simulink model "ssc_lithium_cell_1RC"  (Simulink 7.6)
settings: Solver=ode15s  StartTime=0.0  StopTime=40000  RelTol=1e-3
PreLoadFcn:
  | ssc_lithium_cell_1RC_ini
values from neighbouring files (symbols this model uses):
  C1_LUT = [ ... (first row only)    [ssc_lithium_cell_1RC_ini.m]
  Capacity_LUT = [ ... (first row only)    [ssc_lithium_cell_1RC_ini.m]
  cell_Cp_heat = cell_rho_Cp * cell_volume    (= 810.5328)    [ssc_lithium_cell_1RC_ini.m]
  cell_mass = 1    [ssc_lithium_cell_1RC_ini.m]
  Em_LUT = [ ... (first row only)    [ssc_lithium_cell_1RC_ini.m]
  Qe_init = 15.6845    [ssc_lithium_cell_1RC_ini.m]
  R0_LUT = [ ... (first row only)    [ssc_lithium_cell_1RC_ini.m]
  R1_LUT = [ ... (first row only)    [ssc_lithium_cell_1RC_ini.m]
  SOC_LUT = [0 0.1 0.25 0.5 0.75 0.9 1]'    [ssc_lithium_cell_1RC_ini.m]
  T_init = 20 + 273.15    (= 293.15)    [ssc_lithium_cell_1RC_ini.m]
  Temperature_LUT = [5 20 40] + 273.15    [ssc_lithium_cell_1RC_ini.m]
undefined symbols (not defined in the file or in its folder): sigbuilder_block
libraries: fl_lib x17, nesl_utility x6, LiBatteryElements_lib x4
Description:
  | Lithium Battery Cell - 1 RC Branch Equivalent Circuit
  | 
  | This demo implements a model of a lithium cell using the Simscape language to implement the elements of an equivalent circuit model with one RC branch. For the defining equations and their validation, see T. Huria, M. Ceraolo, J. Gazzarri, R. Jackey. "High Fidelity Electrical Model with Thermal Dependence for Characterization and Simulation of High Power Lithium Battery Cells," IEEE International Electric Vehicle Conference, March 2012.
  | 
  | A simple thermal model is used to model battery temperature. It is assumed that cooling is primarily via convection, and that heating is primarily from battery internal resistance. A battery pack can be modeled by connecting multiple copies of the battery cell block in series.
  | 
  | Copyright 2012 The MathWorks, Inc.
settings Model: Creator=MathWorks  LastModifiedBy=rjackey
settings DataIOCC: SaveOutput=off  SaveTime=off
settings DebuggingCC: SolverPrmCheckMsg=none  StrictBusMsg=Warning

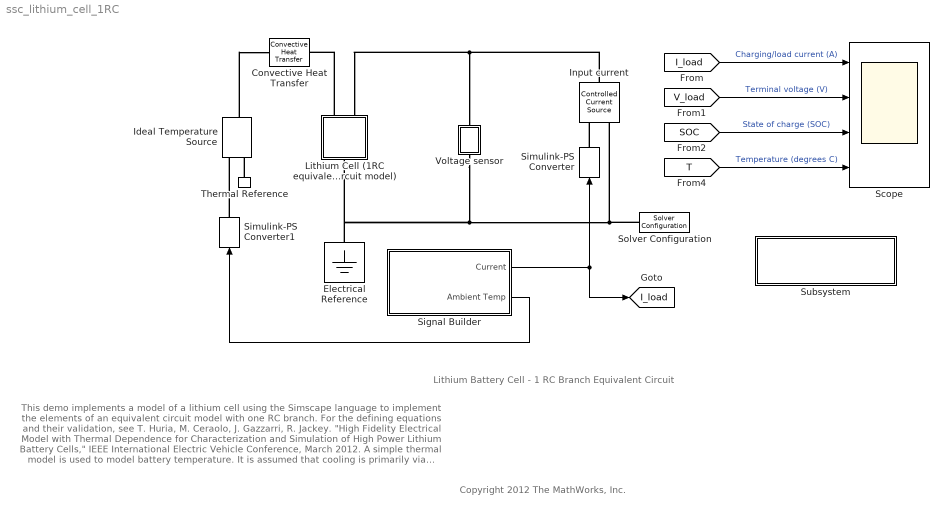
== system ssc_lithium_cell_1RC ==
  note: Lithium Battery Cell - 1 RC Branch Equivalent Circuit
  note: This demo implements a model of a lithium cell using the Simscape language to implement the elements of an equivalent circuit model with one
      | RC branch. For the defining equations and their validation, see T. Huria, M. Ceraolo, J. Gazzarri, R. Jackey. "High Fidelity Electrical Model with
      | Thermal Dependence for Characterization and Simulation of High Power Lithium Battery Cells," IEEE International Electric Vehicle Conference,
      | March 2012. A simple thermal model is used to model battery temperature. It is assumed that cooling is primarily via convection, and that heating
      | is primarily from internal resistance. A battery pack can be modeled by connecting multiple copies of the battery cell block in series.
  note: Copyright 2012 The MathWorks, Inc.
  Convective Heat Transfer : fl_lib/Thermal/Thermal Elements/Convective Heat Transfer  DialogController=NetworkEngine.DynNeDlgSource  SystemSampleTime=-1  area=cell_area m^2  heat_tr_coeff=h_conv W/(m^2 * K)  Q_Log=off  T_Log=off  LocalVarNames=|heat_flow|temperature_diff  LocalVarDescs=|Heat flow (J/s)|Temperature difference (K)  LocalVarLogging=[0 0]
  Electrical Reference : fl_lib/Electrical/Electrical Elements/Electrical Reference  DialogController=NetworkEngine.DynNeDlgSource  SystemSampleTime=-1  i_Log=off  LocalVarNames=|i  LocalVarDescs=|i  LocalVarLogging=[]
  Ideal Temperature Source : fl_lib/Thermal/Thermal Sources/Ideal Temperature Source  DialogController=NetworkEngine.DynNeDlgSource  SystemSampleTime=-1  Q_Log=off  T_Log=off  LocalVarNames=|heat_flow|T_differential  LocalVarDescs=|Heat flow rate through the source (J/s)|Temperature differential across the source (K)  LocalVarLogging=[0 0]
  Input current : fl_lib/Electrical/Electrical Sources/Controlled Current Source  DialogController=NetworkEngine.DynNeDlgSource  SystemSampleTime=-1  i_Log=off  v_Log=off  LocalVarNames=|current|voltage|power  LocalVarDescs=|Current (A)|Voltage (V)|Power (W)  LocalVarLogging=[0 0 0]
  Lithium Cell (1RC equivalent circuit model) : Subsystem  mask{Qe_init=Qe_init, T_init=T_init, Capacity_LUT=Capacity_LUT, Em_LUT=Em_LUT, R0_LUT=R0_LUT, R1_LUT=R1_LUT, C1_LUT=C1_LUT, cell_mass=cell_mass, cell_Cp_heat=cell_Cp_heat, SOC_LUT=SOC_LUT, Temperature_LUT=Temperature_LUT}
      mask prompts: Qe_init "Initial Charge Deficit (A*hr)"; T_init "Initial Cell Temperature (K)"; Capacity_LUT "Capacity (A*hr, 1xN table)"; Em_LUT "Em Open-Circuit Voltage (MxN table)"; R0_LUT "R0: Terminal Resistance (Ohms, MxN table)"; R1_LUT "R1 Resistance (Ohms, MxN table)"; C1_LUT "C1 Capacitance (Farads, MxN table)"; cell_mass "Cell Mass (kg)"; cell_Cp_heat "Cell Specific Heat (J/kg/K)"; SOC_LUT "SOC Table Breakpoints (Mx1 array)"; Temperature_LUT "Temperature Table Breakpoints(K, 1xN array)"
      mask TabNameString: Initial Conditions,Initial Conditions,Electrical,Electrical,Electrical,Electrical,Electrical,Thermal,Thermal,Table Breakpoints,Table Breakpoints
      mask Display:
      | image(imread('battery.jpg'))
      | color('red')
      | port_label('LConn',1,'H')
      | port_label('LConn',2,'+')
      | port_label('RConn',1,'-')
  Scope : Scope  NumInputPorts=4
      settings: TimeRange=40000  YMin=-35~3~0~20  YMax=35~4.5~1~35
  Signal Builder : Subsystem  Tag=STV Subsys  LoadFcn=sigbuilder_block('load');  StartFcn=sigbuilder_block('start');  StopFcn=sigbuilder_block('stop');  ClipboardFcn=sigbuilder_block('clipboard');  mask(Sigbuilder block){}
      mask help: Simulink:masks:SigbuilderBlock_MD
      mask init:
      | if ~strcmp(get_param(bdroot(gcbh),'SimulationStatus'),'stopped') tuvar = sigbuilder_block('maskInit'); end
      settings: CopyFcn=sigbuilder_block('copy');  DeleteFcn=sigbuilder_block('delete');  ModelCloseFcn=sigbuilder_block('modelClose');  PreSaveFcn=sigbuilder_block('preSave');  NameChangeFcn=sigbuilder_block('namechange');  OpenFcn=sigbuilder_block('open',[62.25 82.5 550.5 303 ]);  CloseFcn=sigbuilder_block('close');
      mask Display: plot(0,0,100,100,[10,10,40,40,10],[80,20,20,80,80],[40,10],[50,50], [40,27,10],[65,72,56],[40,25,25,10],[28,28,43,43]);
  Simulink-PS Converter : nesl_utility/Simulink-PS Converter  DialogController=NetworkEngine.DynNeUtilDlgSource  SystemSampleTime=-1  PhysicalDomain=network_engine_domain  LeftPortType=input  RightPortType=output  SubClassName=ps_input  Unit=A  AffineConversion=on  InputFilterTimeConstant=.001  UdotUserProvided=0
  Simulink-PS Converter1 : nesl_utility/Simulink-PS Converter  DialogController=NetworkEngine.DynNeUtilDlgSource  SystemSampleTime=-1  PhysicalDomain=network_engine_domain  LeftPortType=input  RightPortType=output  SubClassName=ps_input  Unit=C  AffineConversion=on  InputFilterTimeConstant=.001  UdotUserProvided=0
  Solver Configuration : nesl_utility/Solver Configuration  DialogController=NetworkEngine.DynNeUtilDlgSource  SystemSampleTime=-1  PhysicalDomain=network_engine_domain  LeftPortType=input  RightPortType=generic  SubClassName=solver  Accelerate=off  Profile=off  ResidualTolerance=1e-9  MaxNonlinIter=3  MaxModeIter=2  DoFixedCost=off  UseLocalSampling=off  DoDC=off  LinearAlgebra=Sparse  LocalSolverSampleTime=.001  LocalSolverChoice=NE_BACKWARD_EULER_ADVANCER  UseLocalSolver=off
  Subsystem : Subsystem
      settings: OpenFcn=open('LiBatteryElements_lib.mdl')
      mask Display: disp('Open the custom\n library used by the\n Lithium Cell block')
  Thermal Reference : fl_lib/Thermal/Thermal Elements/Thermal Reference  DialogController=NetworkEngine.DynNeDlgSource  SystemSampleTime=-1  Q_Log=off  LocalVarNames=|Q  LocalVarDescs=|Q  LocalVarLogging=[]
  Voltage sensor : Subsystem
  tag scope: I_load=global
  wires:
  [SOC] -> Scope/3  "State of charge (SOC)"
  [T] -> Scope/4  "Temperature (degrees C)"
  [I_load] -> Scope/1  "Charging/load current (A)"
  [V_load] -> Scope/2  "Terminal voltage (V)"
  Signal Builder/2(Ambient Temp) -> Simulink-PS Converter1/1
  Signal Builder/1(Current) -> Simulink-PS Converter/1, [I_load]
  connections:
  Electrical Reference/LConn1 -- Lithium Cell (1RC equivalent circuit model)/RConn1 -- Solver Configuration/RConn1 -- Input current/RConn2 -- Voltage sensor/RConn1
  Input current/LConn1 -- Lithium Cell (1RC equivalent circuit model)/LConn2 -- Voltage sensor/LConn1
  Thermal Reference/LConn1 -- Ideal Temperature Source/RConn2
  Ideal Temperature Source/LConn1 -- Convective Heat Transfer/LConn1
  Lithium Cell (1RC equivalent circuit model)/LConn1 -- Convective Heat Transfer/RConn1
  Simulink-PS Converter/RConn1 -- Input current/RConn1
  Simulink-PS Converter1/RConn1 -- Ideal Temperature Source/RConn1

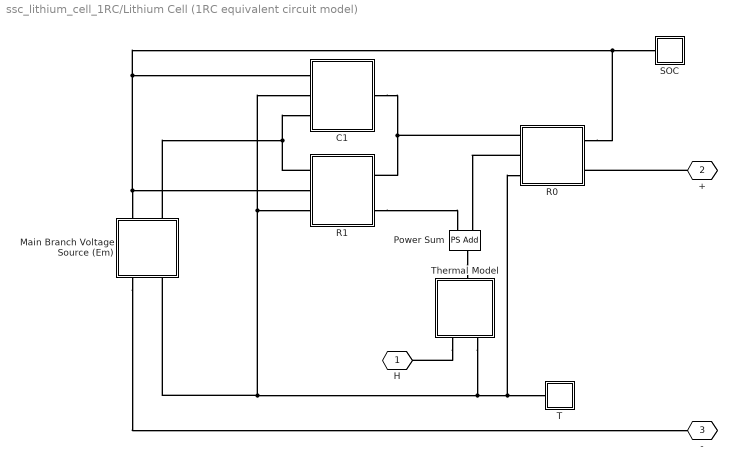
== system ssc_lithium_cell_1RC/Lithium Cell (1RC equivalent circuit model) ==
  " SOC " : Subsystem
  C1 : Subsystem
  Main Branch Voltage Source (Em) : Subsystem
  Power Sum : fl_lib/Physical Signals/Functions/PS Add  DialogController=NetworkEngine.DynNeDlgSource  SystemSampleTime=-1  LocalVarLogging=[]
  R0 : Subsystem
  R1 : Subsystem
  T : Subsystem
  Thermal Model : Subsystem
  H : PMIOPort  Tag=PMCPort  Port=1  Side=Left
  + : PMIOPort  Tag=PMCPort  Port=2  Side=Left
  - : PMIOPort  Tag=PMCPort  Port=3  Side=Right
  connections:
  Main Branch Voltage Source (Em)/LConn1 -- R1/LConn2 -- C1/LConn1 -- " SOC "/LConn1 -- R0/RConn1
  Thermal Model/RConn1 -- H/RConn1
  Main Branch Voltage Source (Em)/RConn1 -- -/RConn1
  +/RConn1 -- R0/RConn2
  R1/LConn1 -- C1/LConn3 -- Main Branch Voltage Source (Em)/LConn2
  R1/RConn2 -- Power Sum/LConn2
  R0/LConn2 -- Power Sum/LConn1
  Main Branch Voltage Source (Em)/RConn2 -- C1/LConn2 -- R1/LConn3 -- Thermal Model/RConn2 -- T/LConn1 -- R0/LConn3
  Power Sum/RConn1 -- Thermal Model/LConn1
  R0/LConn1 -- R1/RConn1 -- C1/RConn1

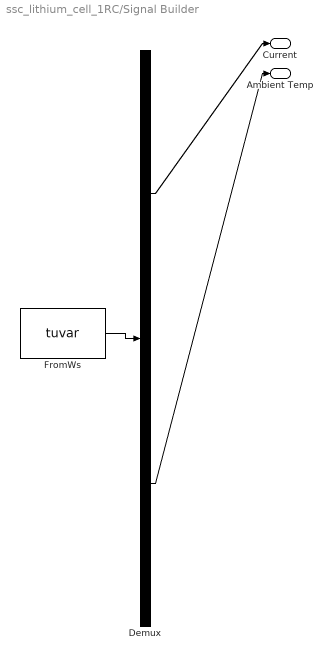
== system ssc_lithium_cell_1RC/Signal Builder ==
  Demux : Demux  Tag=STV Demux  Outputs=2
  FromWs : FromWorkspace  Tag=STV FromWs  VariableName=tuvar  SampleTime=0  SigBuilderData=DataTag0  VnvData=DataTag1
      SigBuilderData=|
      | common.afterFinalStr = 'Extrapolate'
      | common.sampleTime = 0
      | dataSet(1).timeRange = [0 40000]
      | dataSet(1).name = 'Pulse'
      | dataSet(2).timeRange = [0 40000]
      | dataSet(2).name = 'Constant'
      | sbobj.Name = 'Signal Builder'
      | sbobj.Groups(1).Name = 'Pulse'
      | sbobj.Groups(1).Signals(1).Name = 'Current'
      | sbobj.Groups(1).Signals(1).XData = [0 300 300 2100 2100 3600 3600 3960 3960 7200 7200 7560 7560 10800 10800 11160 11160 14400 14400 14760 14760 18000 18000 18360 18360 21600 21600 21960 21960 25200 25200 25560 25560 28800 28800 29160 29160 32400 32400 32760 32760 36000 36000 36360 36360 40000]
      | sbobj.Groups(1).Signals(1).YData = [0 0 31.5 31.5 0 0 -27.625 -27.625 0 0 -27.625 -27.625 0 0 -27.625 -27.625 0 0 -27.625 -27.625 0 0 -27.625 -27.625 0 0 -27.625 -27.625 0 0 -27.625 -27.625 0 0 -27.625 -27.625 0 0 -27.625 -27.625 0 0 -27.625 -27.625 0 0]
      | sbobj.Groups(1).Signals(2).Name = 'Ambient Temp'
      | sbobj.Groups(1).Signals(2).XData = [0 300 300 2100 2100 3600 3600 3960 3960 7200 7200 7560 7560 10800 10800 11160 11160 14400 14400 14760 14760 18000 18000 18360 18360 21600 21600 21960 21960 25200 25200 25560 25560 28800 28800 29160 29160 32400 32400 32760 32760 36000 36000 36360 36360 40000]
      | sbobj.Groups(1).Signals(2).YData = [20 20 20 20 20 20 20 20 20 20 20 20 20 20 20 20 20 20 20 20 20 20 20 20 20 20 20 20 20 20 20 20 20 20 20 20 20 20 20 20 20 20 20 20 20 20]
      | sbobj.Groups(1).TimeRange = [0 40000]
      | sbobj.Groups(2).Name = 'Constant'
      | sbobj.Groups(2).Signals(1).Name = 'Current'
      | sbobj.Groups(2).Signals(1).XData = [0 360 360 9100 9100 11800 11800 28200 33800 40000]
      | sbobj.Groups(2).Signals(1).YData = [0 0 -5 -5 0 0 5 5 0 0]
      | sbobj.Groups(2).Signals(2).Name = 'Ambient Temp'
      | sbobj.Groups(2).Signals(2).XData = [0 360 360 9100 9100 11800 11800 28200 33800 40000]
      | sbobj.Groups(2).Signals(2).YData = [20 20.09 20.09 22.275 22.275 22.95 22.95 27.05 28.45 30]
      | sbobj.Groups(2).TimeRange = [0 40000]
  Current : Outport
  Ambient Temp : Outport  Tag=STV Outport  Port=2
  wires:
  FromWs/1 -> Demux/1
  Demux/1 -> Current/1
  Demux/2 -> Ambient Temp/1

== system ssc_lithium_cell_1RC/Subsystem ==

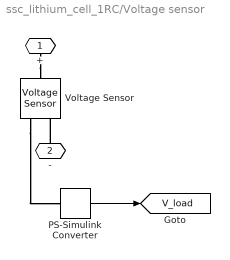
== system ssc_lithium_cell_1RC/Voltage sensor ==
  PS-Simulink Converter : nesl_utility/PS-Simulink Converter  DialogController=NetworkEngine.DynNeUtilDlgSource  SystemSampleTime=-1  PhysicalDomain=network_engine_domain  LeftPortType=input  RightPortType=output  SubClassName=ps_output  Unit=V  AffineConversion=off
  Voltage Sensor : fl_lib/Electrical/Electrical Sensors/Voltage Sensor  DialogController=NetworkEngine.DynNeDlgSource  SystemSampleTime=-1  i1_Log=off  v1_Log=off  LocalVarNames=|i1|v1  LocalVarDescs=|i1|v1  LocalVarLogging=[]
  + : PMIOPort  Port=1  Side=Left
  - : PMIOPort  Port=2  Side=Right
  tag scope: V_load=global
  wires:
  PS-Simulink Converter/1 -> [V_load]
  connections:
  Voltage Sensor/RConn1 -- PS-Simulink Converter/LConn1
  +/RConn1 -- Voltage Sensor/LConn1
  -/RConn1 -- Voltage Sensor/RConn2

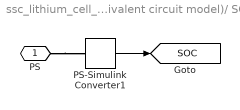
== system ssc_lithium_cell_1RC/Lithium Cell (1RC equivalent circuit model)/ SOC  ==
  PS-Simulink Converter1 : nesl_utility/PS-Simulink Converter  DialogController=NetworkEngine.DynNeUtilDlgSource  SystemSampleTime=-1  PhysicalDomain=network_engine_domain  LeftPortType=input  RightPortType=output  SubClassName=ps_output  Unit=1  AffineConversion=off
  PS : PMIOPort  Port=1  Side=Left
  tag scope: SOC=global
  wires:
  PS-Simulink Converter1/1 -> [SOC]
  connections:
  PS/RConn1 -- PS-Simulink Converter1/LConn1

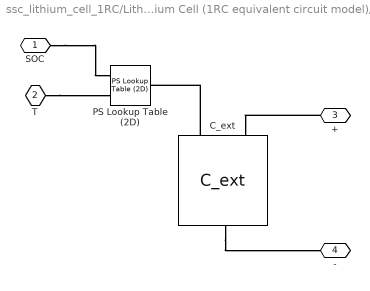
== system ssc_lithium_cell_1RC/Lithium Cell (1RC equivalent circuit model)/C1 ==
  C_ext : LiBatteryElements_lib/C_ext  DialogController=NetworkEngine.DynNeDlgSource  SystemSampleTime=-1  v0=0 V  Cmin=1e-6 F  i_Log=off  v_Log=off  LocalVarNames=|i|v  LocalVarDescs=|i|v  LocalVarLogging=[0 0]
  PS Lookup Table (2D) : fl_lib/Physical Signals/Lookup Tables/PS Lookup Table (2D)  DialogController=NetworkEngine.DynNeDlgSource  SystemSampleTime=-1  x_t=SOC_LUT  y_t=Temperature_LUT  z_t=C1_LUT  interp_method=1  extrap_method=1  dbg=0  LocalVarLogging=[]
  SOC : PMIOPort  Port=1  Side=Left
  T : PMIOPort  Port=2  Side=Left
  + : PMIOPort  Port=3  Side=Left
  - : PMIOPort  Port=4  Side=Right
  connections:
  SOC/RConn1 -- PS Lookup Table (2D)/LConn1
  T/RConn1 -- PS Lookup Table (2D)/LConn2
  C_ext/LConn2 -- PS Lookup Table (2D)/RConn1
  C_ext/RConn1 -- -/RConn1
  +/RConn1 -- C_ext/LConn1

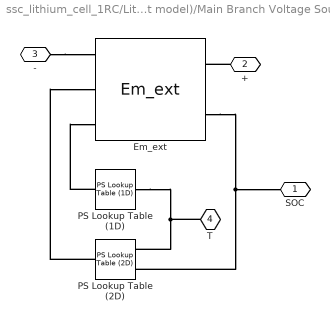
== system ssc_lithium_cell_1RC/Lithium Cell (1RC equivalent circuit model)/Main Branch Voltage Source (Em) ==
  Em_ext : LiBatteryElements_lib/Em_ext  DialogController=NetworkEngine.DynNeDlgSource  SystemSampleTime=-1  Qinit=Qe_init hr*A  i_Log=off  v_Log=off  Qe_Log=off  LocalVarNames=|i|v|Qe  LocalVarDescs=|i|v|Extracted charge  LocalVarLogging=[0 0 0]
  PS Lookup Table (1D) : fl_lib/Physical Signals/Lookup Tables/PS Lookup Table (1D)  DialogController=NetworkEngine.DynNeDlgSource  SystemSampleTime=-1  x_t=Temperature_LUT  y_t=Capacity_LUT  interp_method=1  extrap_method=1  dbg=0  LocalVarLogging=[]
  PS Lookup Table (2D) : fl_lib/Physical Signals/Lookup Tables/PS Lookup Table (2D)  DialogController=NetworkEngine.DynNeDlgSource  SystemSampleTime=-1  x_t=SOC_LUT  y_t=Temperature_LUT  z_t=Em_LUT  interp_method=1  extrap_method=1  dbg=0  LocalVarLogging=[]
  SOC : PMIOPort  Port=1  Side=Left
  + : PMIOPort  Port=2  Side=Left
  - : PMIOPort  Port=3  Side=Right
  T : PMIOPort  Port=4  Side=Right
  connections:
  -/RConn1 -- Em_ext/RConn1
  +/RConn1 -- Em_ext/LConn1
  Em_ext/LConn2 -- SOC/RConn1 -- PS Lookup Table (2D)/LConn1
  PS Lookup Table (2D)/RConn1 -- Em_ext/RConn2
  PS Lookup Table (1D)/LConn1 -- PS Lookup Table (2D)/LConn2 -- T/RConn1
  PS Lookup Table (1D)/RConn1 -- Em_ext/RConn3

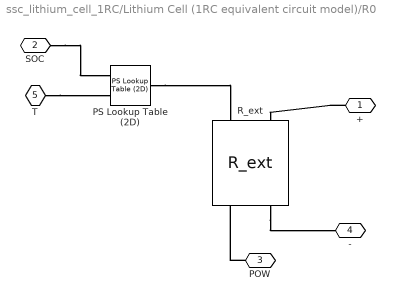
== system ssc_lithium_cell_1RC/Lithium Cell (1RC equivalent circuit model)/R0 ==
  PS Lookup Table (2D) : fl_lib/Physical Signals/Lookup Tables/PS Lookup Table (2D)  DialogController=NetworkEngine.DynNeDlgSource  SystemSampleTime=-1  x_t=SOC_LUT  y_t=Temperature_LUT  z_t=R0_LUT  interp_method=1  extrap_method=1  dbg=0  LocalVarLogging=[]
  R_ext : LiBatteryElements_lib/R_ext  DialogController=NetworkEngine.DynNeDlgSource  SystemSampleTime=-1  Rmin=0 Ohm  i_Log=off  v_Log=off  LocalVarNames=|i|v  LocalVarDescs=|i|v  LocalVarLogging=[0 0]
  + : PMIOPort  Port=1  Side=Left
  SOC : PMIOPort  Port=2  Side=Right
  POW : PMIOPort  Port=3  Side=Left
  - : PMIOPort  Port=4  Side=Right
  T : PMIOPort  Port=5  Side=Left
  connections:
  T/RConn1 -- PS Lookup Table (2D)/LConn2
  +/RConn1 -- R_ext/LConn1
  R_ext/RConn1 -- -/RConn1
  POW/RConn1 -- R_ext/RConn2
  PS Lookup Table (2D)/RConn1 -- R_ext/LConn2
  SOC/RConn1 -- PS Lookup Table (2D)/LConn1

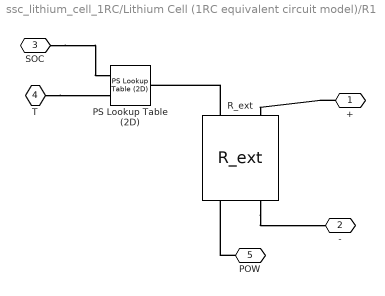
== system ssc_lithium_cell_1RC/Lithium Cell (1RC equivalent circuit model)/R1 ==
  PS Lookup Table (2D) : fl_lib/Physical Signals/Lookup Tables/PS Lookup Table (2D)  DialogController=NetworkEngine.DynNeDlgSource  SystemSampleTime=-1  x_t=SOC_LUT  y_t=Temperature_LUT  z_t=R1_LUT  interp_method=1  extrap_method=1  dbg=0  LocalVarLogging=[]
  R_ext : LiBatteryElements_lib/R_ext  DialogController=NetworkEngine.DynNeDlgSource  SystemSampleTime=-1  Rmin=0 Ohm  i_Log=off  v_Log=off  LocalVarNames=|i|v  LocalVarDescs=|i|v  LocalVarLogging=[0 0]
  + : PMIOPort  Port=1  Side=Left
  - : PMIOPort  Port=2  Side=Right
  SOC : PMIOPort  Port=3  Side=Left
  T : PMIOPort  Port=4  Side=Left
  POW : PMIOPort  Port=5  Side=Right
  connections:
  SOC/RConn1 -- PS Lookup Table (2D)/LConn1
  T/RConn1 -- PS Lookup Table (2D)/LConn2
  R_ext/LConn2 -- PS Lookup Table (2D)/RConn1
  POW/RConn1 -- R_ext/RConn2
  R_ext/RConn1 -- -/RConn1
  +/RConn1 -- R_ext/LConn1

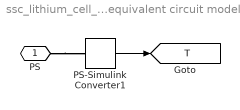
== system ssc_lithium_cell_1RC/Lithium Cell (1RC equivalent circuit model)/T ==
  PS-Simulink Converter1 : nesl_utility/PS-Simulink Converter  DialogController=NetworkEngine.DynNeUtilDlgSource  SystemSampleTime=-1  PhysicalDomain=network_engine_domain  LeftPortType=input  RightPortType=output  SubClassName=ps_output  Unit=C  AffineConversion=on
  PS : PMIOPort  Port=1  Side=Left
  tag scope: T=global
  wires:
  PS-Simulink Converter1/1 -> [T]
  connections:
  PS/RConn1 -- PS-Simulink Converter1/LConn1

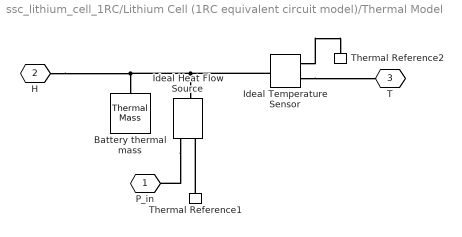
== system ssc_lithium_cell_1RC/Lithium Cell (1RC equivalent circuit model)/Thermal Model ==
  Battery thermal mass : fl_lib/Thermal/Thermal Elements/Thermal Mass  DialogController=NetworkEngine.DynNeDlgSource  SystemSampleTime=-1  mass=cell_mass kg  sp_heat=cell_Cp_heat J/kg/K  init_temp=T_init K  Q_Log=off  LocalVarNames=|heat_flow|temperature  LocalVarDescs=|Heat flow (J/s)|Mass temperature (K)  LocalVarLogging=[0 0]
  Ideal Temperature Sensor : fl_lib/Thermal/Thermal Sensors/Ideal Temperature Sensor  DialogController=NetworkEngine.DynNeDlgSource  SystemSampleTime=-1  Qs_Log=off  Ts_Log=off  LocalVarNames=|Qs|Ts  LocalVarDescs=|Qs|Ts  LocalVarLogging=[]
  Ideal Heat Flow Source : fl_lib/Thermal/Thermal Sources/Ideal Heat Flow Source  DialogController=NetworkEngine.DynNeDlgSource  SystemSampleTime=-1  Q_Log=off  T_Log=off  LocalVarNames=|heat_flow|T_differential  LocalVarDescs=|Heat flow through the source (J/s)|Temperature differential across the source (K)  LocalVarLogging=[0 0]
  Thermal Reference1 : fl_lib/Thermal/Thermal Elements/Thermal Reference  DialogController=NetworkEngine.DynNeDlgSource  SystemSampleTime=-1  Q_Log=off  LocalVarNames=|Q  LocalVarDescs=|Q  LocalVarLogging=[]
  Thermal Reference2 : fl_lib/Thermal/Thermal Elements/Thermal Reference  DialogController=NetworkEngine.DynNeDlgSource  SystemSampleTime=-1  Q_Log=off  LocalVarNames=|Q  LocalVarDescs=|Q  LocalVarLogging=[]
  P_in : PMIOPort  Tag=PMCPort  Port=1  Side=Left
  H : PMIOPort  Tag=PMCPort  Port=2  Side=Right
  T : PMIOPort  Tag=PMCPort  Port=3  Side=Right
  connections:
  Ideal Temperature Sensor/RConn1 -- Thermal Reference2/LConn1
  Ideal Temperature Sensor/RConn2 -- T/RConn1
  Thermal Reference1/LConn1 -- Ideal Heat Flow Source/RConn2
  Ideal Temperature Sensor/LConn1 -- H/RConn1 -- Battery thermal mass/LConn1 -- Ideal Heat Flow Source/LConn1
  Ideal Heat Flow Source/RConn1 -- P_in/RConn1
